simulink model "hummel_and_hubbard"  (R2021b)
settings: Solver=VariableStepAuto  StartTime=0.0  StopTime=10.0  RelTol=1e-3
values from neighbouring files (symbols this model uses):
  amb = evalin( 'base', 'amb')    [flatball_6dof_eqom.m]
  C = evalin( 'base', 'C')    [flatball_6dof_eqom.m]
  disc = evalin( 'base', 'disc')    [flatball_6dof_eqom.m]    (also in flatball_6dof_init.m = struct; flatball_init_disc_params.m = struct)
  Y0 = [0 0 -1, 0 15*C.DEG2RAD 0, 15 0 0, 0 0 (2*15*0.29/disc.d)]    [flatball_6dof_eqom.m]
libraries: simulink x4, aerolibanim x2, aerolibnav x2, matrix_library x2, mspfiltlib x1
(part 1 of 3)
settings Model: Creator=schae  LastModifiedBy=schae

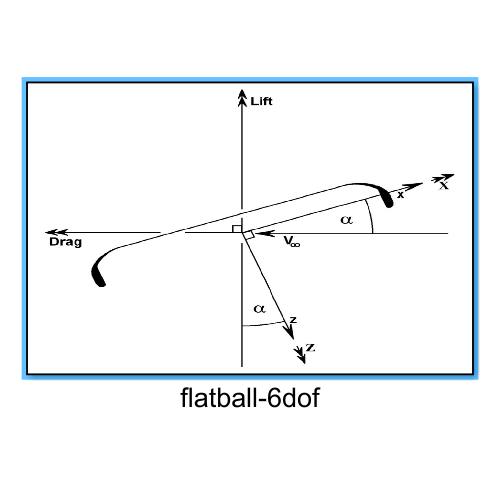
[thumbnail: Simulink's stored preview of the top-level diagram]
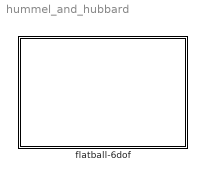
== system hummel_and_hubbard ==
  flatball-6dof : Subsystem
      mask Display: image('C:\.local\desktop\misc.protolabs\flatball-aero-ssl\arxiv\img\screenshots\flatball-6dof.png'); % Use "Edit Image" on toolstrip to change.

== system hummel_and_hubbard/flatball-6dof ==
  Integrator4 : Integrator  InitialConditionSource=external
  Selector : Selector  Commented=through  InputPortWidth=12  IndexOptions=Index vector (dialog)  Indices=[1 2 3 7 8 9 4 5 6 10 11 12]  OutputSizes=1
  Selector1 : Selector  Commented=through  InputPortWidth=12  IndexOptions=Index vector (dialog)  Indices=[1 2 3 7 8 9 4 5 6 10 11 12]  OutputSizes=1
  X0_desired : Constant  Value=Y0
  calc-F-M : Subsystem
  calc-Xdot : Subsystem
  lab : Subsystem
  wires:
  calc-F-M/2(M) -> [M]
  calc-F-M/1(F) -> [F]
  [X] -> Selector/1
  [F] -> calc-Xdot/2(F)
  calc-Xdot/1(Xdot) -> [dXdt], Integrator4/1
  X0_desired/1 -> Selector1/1
  [M] -> calc-Xdot/3(M)
  Integrator4/1 -> [X]  "X"
  [dXdt] -> lab/1(dYdt)
  [X] -> lab/2(Y)
  Selector/1 -> calc-F-M/1(X), calc-Xdot/1(X)
  Selector1/1 -> Integrator4/2

== system hummel_and_hubbard/flatball-6dof/calc-F-M ==
  X : Inport
  From1 : From  Commented=on  GotoTag=X
  From10 : From  Commented=on  GotoTag=F
  From11 : From  Commented=on  GotoTag=M
  From5 : From  Commented=on  GotoTag=alpha
  From6 : From  Commented=on  GotoTag=T
  From9 : From  Commented=on  GotoTag=wD
  calc-F : Subsystem
  calc-M : Subsystem
  calc-alpha : Subsystem
  lab : Subsystem  Commented=on
  rotations : Subsystem
  F : Outport
  M : Outport  Port=2
  wires:
  From1/1 -> lab/1(X)
  From10/1 -> lab/5(F)
  From6/1 -> lab/2(T)
  X/1 -> calc-M/1(X), calc-alpha/1(X), rotations/1(X), calc-F/1(X)
  [T] -> calc-M/2(T_c_N), calc-F/2(T_c_N)
  From9/1 -> lab/3(wD)
  [T] -> calc-alpha/2(T_c_N)
  rotations/1(T_c_N) -> [T]
  [alpha] -> calc-F/3(alpha), calc-M/4(alpha)
  From11/1 -> lab/6(M)
  rotations/2(wD_N) -> [wD]
  [wD] -> calc-M/3(wD_N_inN)
  calc-alpha/1(alpha) -> [alpha]
  From5/1 -> lab/4(alpha)
  calc-F/1(F) -> F/1  "F"
  calc-M/1(M) -> M/1  "M"

== system hummel_and_hubbard/flatball-6dof/calc-Xdot ==
  X : Inport
  F : Inport  Port=2
  M : Inport  Port=3
  Demux1 : Demux  Outputs=[1 1 1 1 1 1 1 1 1 1 1 1]
  Mux : Mux  Inputs=2
  Reshape : Reshape
  Selector : Selector  InputPortWidth=12  IndexOptions=Index vector (dialog)  Indices=[1 2 3 7 8 9 4 5 6 10 11 12]  OutputSizes=1
  Terminator{,1..11} (12 alike) : Terminator
  calc-THdot : MATLAB Function  TreatAsAtomicUnit=on
  calc-Xdot : MATLAB Function  TreatAsAtomicUnit=on
  Xdot : Outport
  wires:
  calc-Xdot/1(Xdot) -> Mux/1  "Xdot"
  Mux/1 -> Selector/1
  X/1 -> calc-THdot/1(X), calc-Xdot/1(X), [X]
  M/1 -> calc-THdot/2(M)
  F/1 -> calc-Xdot/2(F)
  calc-THdot/1(THdot) -> Mux/2  "THdot"
  Demux1/1 -> Terminator/1  "x"
  Demux1/2 -> Terminator1/1  "y"
  Demux1/3 -> Terminator2/1  "z"
  Demux1/6 -> Terminator5/1  "w"
  Demux1/5 -> Terminator4/1  "v"
  Demux1/4 -> Terminator3/1  "u"
  Demux1/10 -> Terminator9/1  "phidt"
  Demux1/11 -> Terminator10/1  "thetadt"
  Demux1/12 -> Terminator11/1  "psidt"
  Demux1/9 -> Terminator8/1  "psi"
  Demux1/8 -> Terminator7/1  "theta"
  Demux1/7 -> Terminator6/1  "phi"
  [X] -> Reshape/1
  Reshape/1 -> Demux1/1
  Selector/1 -> Xdot/1

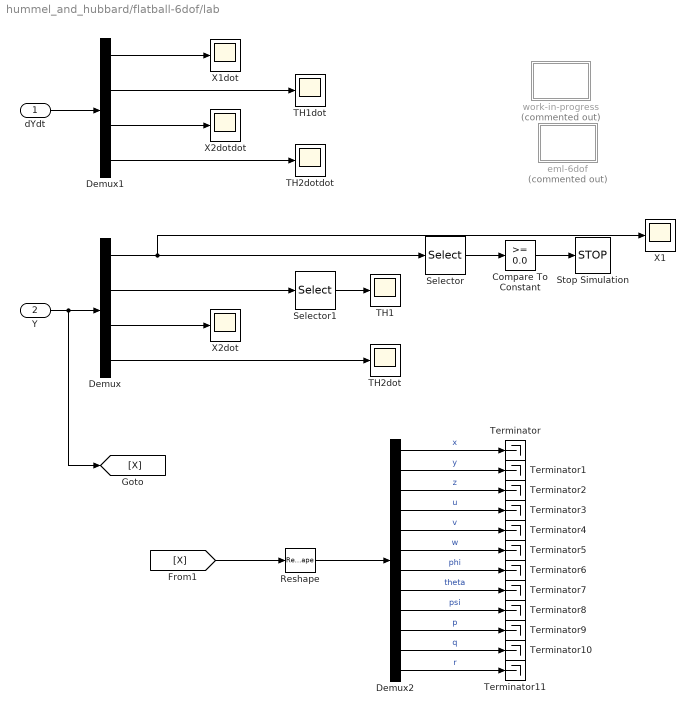
== system hummel_and_hubbard/flatball-6dof/lab ==
  dYdt : Inport
  Y : Inport  Port=2
  Compare To Constant : simulink/Logic and Bit Operations/Compare To Constant  relop=>=  const=0.0  OutDataTypeStr=boolean
  Demux : Demux  Outputs=[3 3 3 3]
  Demux1 : Demux  Outputs=[3 3 3 3]
  Demux2 : Demux  Outputs=[1 1 1 1 1 1 1 1 1 1 1 1]
  Reshape : Reshape
  Selector : Selector  InputPortWidth=3  IndexOptions=Index vector (dialog)  Indices=[3]  OutputSizes=1
  Selector1 : Selector  InputPortWidth=3  IndexOptions=Index vector (dialog)  Indices=[1 2]  OutputSizes=1
  Stop Simulation : Stop
  TH1 : Scope
  TH1dot : Scope
  TH2dot : Scope
  TH2dotdot : Scope
  Terminator{,1..11} (12 alike) : Terminator
  X1 : Scope
  X1dot : Scope
  X2dot : Scope
  X2dotdot : Scope
  eml-6dof : Subsystem  Commented=on
  work-in-progress : Subsystem  Commented=on
  wires:
  Demux2/4 -> Terminator3/1  "u"
  Demux2/3 -> Terminator2/1  "z"
  Demux2/2 -> Terminator1/1  "y"
  Demux2/6 -> Terminator5/1  "w"
  Demux2/1 -> Terminator/1  "x"
  Demux2/5 -> Terminator4/1  "v"
  Demux2/8 -> Terminator7/1  "theta"
  Demux2/7 -> Terminator6/1  "phi"
  Demux2/9 -> Terminator8/1  "psi"
  Demux2/10 -> Terminator9/1  "p"
  Demux2/11 -> Terminator10/1  "q"
  [X] -> Reshape/1
  Reshape/1 -> Demux2/1
  Demux2/12 -> Terminator11/1  "r"
  Compare To Constant/1 -> Stop Simulation/1
  Selector/1 -> Compare To Constant/1
  Selector1/1 -> TH1/1
  Y/1 -> Demux/1, [X]
  Demux/1 -> Selector/1, X1/1
  Demux/2 -> Selector1/1
  Demux/3 -> X2dot/1
  Demux/4 -> TH2dot/1
  dYdt/1 -> Demux1/1
  Demux1/1 -> X1dot/1
  Demux1/2 -> TH1dot/1
  Demux1/4 -> TH2dotdot/1
  Demux1/3 -> X2dotdot/1

== system hummel_and_hubbard/flatball-6dof/calc-F-M/calc-F ==
  X : Inport
  T_c_N : Inport  Port=2
  alpha : Inport  Port=3
  Fg_N : Constant  Value=[0 0 disc.m*amb.g]'
  Terminator{,1..3} (4 alike) : Terminator
  X-to-vel : MATLAB Function  TreatAsAtomicUnit=on
  aero-coeff : Subsystem
  calc-F : MATLAB Function  TreatAsAtomicUnit=on
  q-inf : Subsystem
  F : Outport
  wires:
  X-to-vel/1(vel) -> calc-F/1(vel)  "vel"
  X/1 -> q-inf/1(X), X-to-vel/1(X)
  T_c_N/1 -> calc-F/2(T_c_N)
  Fg_N/1 -> calc-F/3(Fg_N)
  calc-F/1(F) -> F/1  "F"
  q-inf/1(q-inf-S) -> calc-F/6(q_inf_times_S)
  alpha/1 -> aero-coeff/1(alpha)
  aero-coeff/1(Cl) -> calc-F/4(CLift)
  aero-coeff/2(Cd) -> calc-F/5(CDrag)
  q-inf/2(q-inf-S-d) -> Terminator/1
  calc-F/2(lift) -> Terminator1/1  "lift"
  calc-F/3(drag) -> Terminator2/1  "drag"
  calc-F/4(vmag) -> Terminator3/1  "v_inf"

== system hummel_and_hubbard/flatball-6dof/calc-F-M/calc-M ==
  X : Inport
  T_c_N : Inport  Port=2
  wD_N_inN : Inport  Port=3
  alpha : Inport  Port=4
  Terminator{,1..6} (7 alike) : Terminator
  X-to-vel : MATLAB Function  TreatAsAtomicUnit=on
  aero-coeff : Subsystem
  calc-M : MATLAB Function  TreatAsAtomicUnit=on
  internals : MATLAB Function  TreatAsAtomicUnit=on
  q-inf : Subsystem
  M : Outport
  wires:
  alpha/1 -> aero-coeff/1(alpha)
  calc-M/1(M) -> M/1  "M"
  T_c_N/1 -> calc-M/2(T_c_N), internals/2(T_c_N)
  X/1 -> X-to-vel/1(X), internals/1(X), q-inf/1(X)
  X-to-vel/1(vel) -> calc-M/1(vel)
  q-inf/2(q-inf-S-d) -> calc-M/4(q_inf_times_Sd)
  aero-coeff/1(Cm) -> calc-M/5(CMpitch)
  wD_N_inN/1 -> internals/3(wD_N_inN), calc-M/3(wD_N_inN)
  q-inf/1(q-inf-S) -> Terminator/1
  calc-M/2(p) -> Terminator1/1  "p"
  calc-M/3(q) -> Terminator2/1  "q"
  calc-M/4(r) -> Terminator3/1  "r"
  internals/3(E_rot) -> Terminator6/1  "E_rot"
  internals/2(E_trans) -> Terminator5/1  "E_trans"
  internals/1(AdvR) -> Terminator4/1  "AdvR"

== system hummel_and_hubbard/flatball-6dof/calc-F-M/calc-alpha ==
  X : Inport
  T_c_N : Inport  Port=2
  calc-alpha : MATLAB Function  TreatAsAtomicUnit=on
  alpha : Outport
  wires:
  calc-alpha/1(alpha) -> alpha/1  "alpha"
  X/1 -> calc-alpha/1(X)
  T_c_N/1 -> calc-alpha/2(T_c_N)

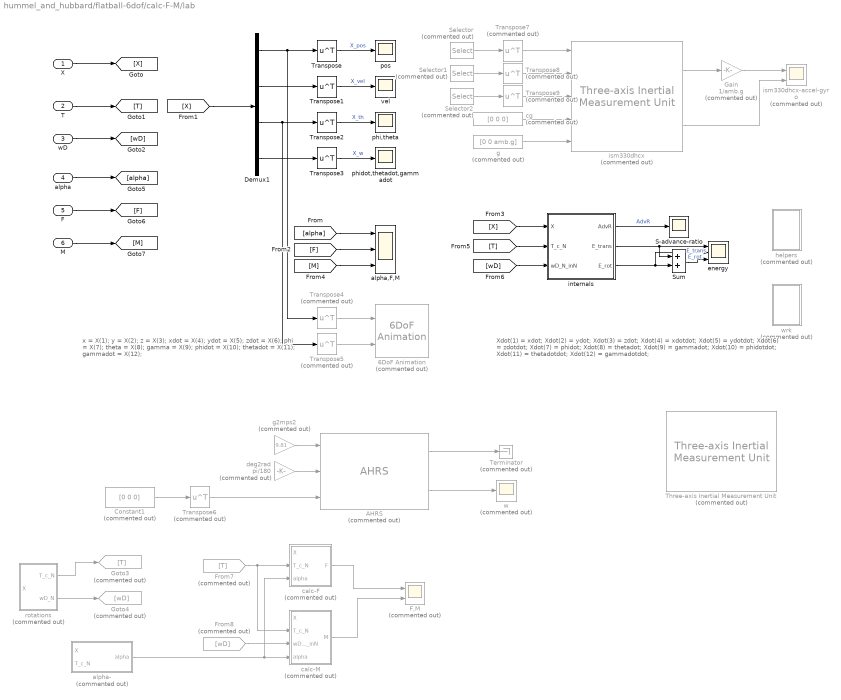
== system hummel_and_hubbard/flatball-6dof/calc-F-M/lab ==
  note: x = X(1); y = X(2); z = X(3);
      | xdot = X(4); ydot = X(5); zdot = X(6);
      |
      | phi = X(7); theta = X(8); gamma = X(9);
      | phidot = X(10); thetadot = X(11); gammadot = X(12);
  note: Xdot(1) = xdot; Xdot(2) = ydot; Xdot(3) = zdot;
      | Xdot(4) = xdotdot; Xdot(5) = ydotdot; Xdot(6) = zdotdot;
      |
      | Xdot(7) = phidot; Xdot(8) = thetadot; Xdot(9) = gammadot;
      | Xdot(10) = phidotdot; Xdot(11) = thetadotdot; Xdot(12) = gammadotdot;
  X : Inport
  T : Inport  Port=2
  wD : Inport  Port=3
  alpha : Inport  Port=4
  F : Inport  Port=5
  M : Inport  Port=6
  6DoF Animation : aerolibanim/6DoF Animation  Commented=on  u1=[-20 50 -20 50 -20 5]  u2=0.1  u3=1.0  u4=[-1 -1 -1]  u5=Fixed position  u6=[-200 -20 -10]  u7=10  u8=on
  AHRS : mspfiltlib/AHRS  Commented=on  DispRefFrame=ENU  DecimationFactor=1  InitialProcessNoise=ahrsfilter.defaultProcessNoise  OrientationFormat=Rotation matrix  SimulateUsing=Interpreted execution  AccelerometerNoise=0.0001924722  GyroscopeNoise=9.1385e-5  MagnetometerNoise=0.1  GyroscopeDriftNoise=3.0462e-13  LinearAccelerationNoise=0.0096236100000000012  MagneticDisturbanceNoise=0.5  LinearAccelerationDecayFactor=0.5  MagneticDisturbanceDecayFactor=0.5  ExpectedMagneticFieldStrength=50
      settings: SourceProductBaseCode=TF,NV
  Constant1 : Constant  Commented=on  Value=[0 0 0]
  Demux1 : Demux  Outputs=[3 3 3 3]
  F,M : Scope  Commented=on  NumInputPorts=2
  From7 : From  Commented=on  GotoTag=T
  From8 : From  Commented=on  GotoTag=wD
  Gain : Gain  Commented=on  Gain=1/amb.g
  Goto3 : Goto  Commented=on  GotoTag=T
  Goto4 : Goto  Commented=on  GotoTag=wD
  S-advance-ratio : Scope
  Selector : Selector  Commented=on  InputPortWidth=12  IndexOptions=Index vector (dialog)  Indices=[4 5 6]  OutputSizes=1
  Selector1 : Selector  Commented=on  InputPortWidth=12  IndexOptions=Index vector (dialog)  Indices=[7 8 9]  OutputSizes=1
  Selector2 : Selector  Commented=on  InputPortWidth=12  IndexOptions=Index vector (dialog)  Indices=[7 8 9]  OutputSizes=1
  Sum : Sum  Inputs=2
  Terminator : Terminator  Commented=on
  Three-axis Inertial Measurement Unit : aerolibnav/Three-axis Inertial Measurement Unit  Commented=on  units=Metric (MKS)  imu=[0 0 0]  i_Ts=0  dtype_a=on  w_a=190  z_a=0.707  a_sf_cc=[1 0 0; 0 1 0; 0 0 1]  a_bias=[0 0 0]  a_sat="[-inf  -inf  -inf  inf inf inf]"  dtype_g=on  w_g=190  z_g=0.707  g_sf_cc=[1 0 0; 0 1 0; 0 0 1]  g_bias=[0 0 0]  g_sens=[0 0 0]  g_sat="[-inf  -inf  -inf  inf inf inf]"  i_rand=on  i_seeds=[23093 23094 23095 23096 23097 23098]  i_pow=[0.001 0.001 0.001 0.0001 0.0001 0.0001]
  Transpose{,1..3} (4 alike) : Math  Operator=transpose  SaturateOnIntegerOverflow=on
  Transpose{4..9} (6 alike) : Math  Commented=on  Operator=transpose  SaturateOnIntegerOverflow=on
  alpha,F,M : Scope  NumInputPorts=3
  alpha- : MATLAB Function  Commented=on  TreatAsAtomicUnit=on
  calc-F : Subsystem  Commented=on
  calc-M : Subsystem  Commented=on
  cg : Constant  Commented=on  Value=[0 0 0]
  deg2rad : Gain  Commented=on  Gain=pi/180
  energy : Scope  NumInputPorts=3
  g : Constant  Commented=on  Value=[0 0 amb.g]
  g2mps2 : Gain  Commented=on  Gain=9.81
  helpers : Subsystem  Commented=on
  internals : MATLAB Function  TreatAsAtomicUnit=on
  ism330dhcx : aerolibnav/Three-axis Inertial Measurement Unit  Commented=on  units=Metric (MKS)  imu=[-2e-3 1e-3 -5e-3]  i_Ts=0  dtype_a=on  w_a=190  z_a=0.707  a_sf_cc=[1 0 0; 0 1 0; 0 0 1]  a_bias=[0 0 0]  a_sat="[-inf  -inf  -inf  inf inf inf]"  dtype_g=on  w_g=190  z_g=0.707  g_sf_cc=[1 0 0; 0 1 0; 0 0 1]  g_bias=[0 0 0]  g_sens=[0 0 0]  g_sat="[-inf  -inf  -inf  inf inf inf]"  i_rand=on  i_seeds=[23093 23094 23095 23096 23097 23098]  i_pow=[0.001 0.001 0.001 0.0001 0.0001 0.0001]
  ism330dhcx-accel-gyro : Scope  Commented=on  NumInputPorts=2
  phi,theta : Scope
  phidot,thetadot,gammadot : Scope
  pos : Scope
  rotations : Subsystem  Commented=on
  vel : Scope
  w : Scope  Commented=on
  wrk : Subsystem  Commented=on
  wires:
  From7/1 -> calc-M/2(T_c_N), calc-F/2(T_c_N)
  alpha-/1(alpha) -> calc-F/3(alpha), calc-M/4(alpha)
  From8/1 -> calc-M/3(wD_N_inN)
  calc-M/1(M) -> F,M/2
  calc-F/1(F) -> F,M/1
  rotations/1(T_c_N) -> Goto3/1
  rotations/2(wD_N) -> Goto4/1
  internals/3(E_rot) -> Sum/2, energy/2  "E_rot"
  [wD] -> internals/3(wD_N_inN)
  internals/1(AdvR) -> S-advance-ratio/1  "AdvR"
  [T] -> internals/2(T_c_N)
  Sum/1 -> energy/3
  [X] -> internals/1(X)
  internals/2(E_trans) -> Sum/1, energy/1  "E_trans"
  Demux1/4 -> Transpose3/1
  Demux1/3 -> Transpose5/1, Transpose2/1
  Demux1/1 -> Transpose4/1, Transpose/1
  Demux1/2 -> Transpose1/1
  [X] -> Demux1/1
  X/1 -> [X]
  T/1 -> [T]
  wD/1 -> [wD]
  F/1 -> [F]
  alpha/1 -> [alpha]
  M/1 -> [M]
  [alpha] -> alpha,F,M/1
  [F] -> alpha,F,M/2
  [M] -> alpha,F,M/3
  Transpose/1 -> pos/1  "X_pos"
  Transpose1/1 -> vel/1  "X_vel"
  Transpose2/1 -> phi,theta/1  "X_th"
  Transpose3/1 -> phidot,thetadot,gammadot/1  "X_w"
  Transpose4/1 -> 6DoF Animation/1
  Transpose5/1 -> 6DoF Animation/2
  Transpose6/1 -> AHRS/3
  Constant1/1 -> Transpose6/1
  AHRS/2 -> w/1
  g2mps2/1 -> AHRS/1
  deg2rad/1 -> AHRS/2
  AHRS/1 -> Terminator/1
  Transpose7/1 -> ism330dhcx/1
  Selector/1 -> Transpose7/1
  g/1 -> ism330dhcx/5
  Transpose8/1 -> ism330dhcx/2
  cg/1 -> ism330dhcx/4
  ism330dhcx/1 -> Gain/1
  Transpose9/1 -> ism330dhcx/3
  Selector1/1 -> Transpose8/1
  Selector2/1 -> Transpose9/1
  Gain/1 -> ism330dhcx-accel-gyro/1
  ism330dhcx/2 -> ism330dhcx-accel-gyro/2

== system hummel_and_hubbard/flatball-6dof/calc-F-M/rotations ==
  X : Inport
  MatrixMultiply3 : Product  Multiplication=Matrix(*)
  Transpose : Math  Operator=transpose  SaturateOnIntegerOverflow=on
  Transpose1 : Math  Operator=transpose  SaturateOnIntegerOverflow=on
  X-to-T_c_N : MATLAB Function  TreatAsAtomicUnit=on
  X-to-wD_N_inC : MATLAB Function  TreatAsAtomicUnit=on
  T_c_N : Outport
  wD_N : Outport  Port=2
  wires:
  X-to-T_c_N/1(T_c_N) -> Transpose1/1, T_c_N/1
  Transpose1/1 -> MatrixMultiply3/1
  X-to-wD_N_inC/1(wD_N_inC) -> Transpose/1
  Transpose/1 -> MatrixMultiply3/2
  MatrixMultiply3/1 -> wD_N/1
  X/1 -> X-to-wD_N_inC/1(X), X-to-T_c_N/1(X)

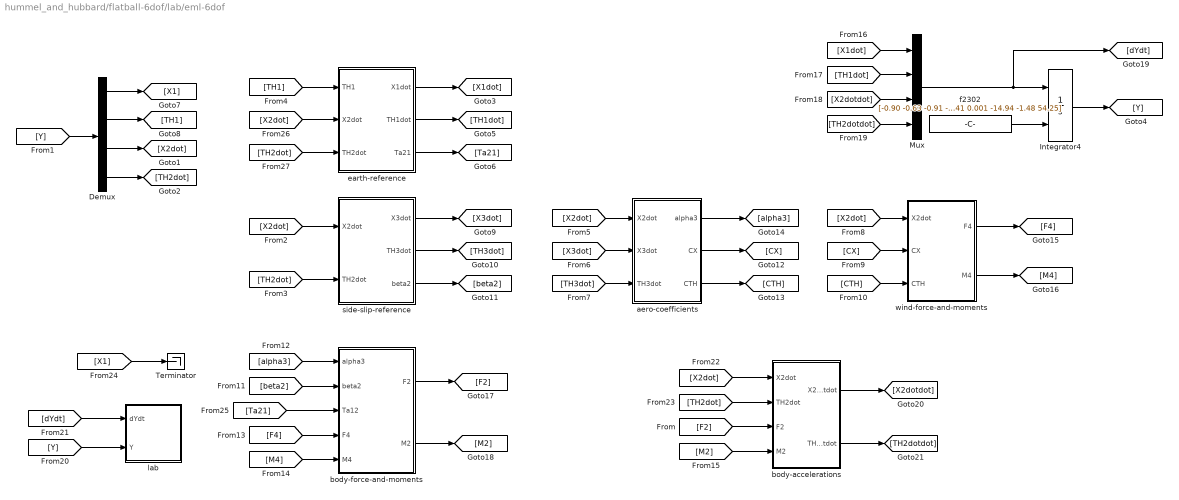
== system hummel_and_hubbard/flatball-6dof/lab/eml-6dof ==
  Demux : Demux  Outputs=[3 3 3 3]
  Integrator4 : Integrator  InitialConditionSource=external
  Mux : Mux
  Terminator : Terminator
  aero-coefficients : MATLAB Function  TreatAsAtomicUnit=on
  body-accelerations : MATLAB Function  TreatAsAtomicUnit=on
  body-force-and-moments : MATLAB Function  TreatAsAtomicUnit=on
  earth-reference : MATLAB Function  TreatAsAtomicUnit=on
  f2302 : Constant  Value=[-0.90 -0.63 -0.91 -0.07 0.21 5.03 13.42 -0.41 0.001 -14.94 -1.48 54.25]
  lab : Subsystem
  side-slip-reference : MATLAB Function  TreatAsAtomicUnit=on
  wind-force-and-moments : MATLAB Function  TreatAsAtomicUnit=on
  wires:
  earth-reference/1(X1dot) -> [X1dot]
  earth-reference/2(TH1dot) -> [TH1dot]
  earth-reference/3(Ta21) -> [Ta21]
  [Y] -> Demux/1
  Demux/1 -> [X1]
  Demux/2 -> [TH1]
  Demux/3 -> [X2dot]
  Demux/4 -> [TH2dot]
  [X2dot] -> side-slip-reference/1(X2dot)
  [TH2dot] -> side-slip-reference/2(TH2dot)
  side-slip-reference/1(X3dot) -> [X3dot]
  side-slip-reference/2(TH3dot) -> [TH3dot]
  side-slip-reference/3(beta2) -> [beta2]
  [TH1] -> earth-reference/1(TH1)
  [X2dot] -> aero-coefficients/1(X2dot)
  [X3dot] -> aero-coefficients/2(X3dot)
  [TH3dot] -> aero-coefficients/3(TH3dot)
  aero-coefficients/3(CTH) -> [CTH]
  aero-coefficients/2(CX) -> [CX]
  aero-coefficients/1(alpha3) -> [alpha3]
  [X2dot] -> wind-force-and-moments/1(X2dot)
  [CX] -> wind-force-and-moments/2(CX)
  [CTH] -> wind-force-and-moments/3(CTH)
  [beta2] -> body-force-and-moments/2(beta2)
  [alpha3] -> body-force-and-moments/1(alpha3)
  wind-force-and-moments/1(F4) -> [F4]
  wind-force-and-moments/2(M4) -> [M4]
  [F4] -> body-force-and-moments/4(F4)
  [M4] -> body-force-and-moments/5(M4)
  body-force-and-moments/1(F2) -> [F2]
  body-force-and-moments/2(M2) -> [M2]
  [TH2dotdot] -> Mux/4
  Mux/1 -> Integrator4/1, [dYdt]
  [TH1dot] -> Mux/2
  [X1dot] -> Mux/1
  f2302/1 -> Integrator4/2
  [X2dotdot] -> Mux/3
  Integrator4/1 -> [Y]
  [dYdt] -> lab/1(dYdt)
  [Y] -> lab/2(Y)
  [F2] -> body-accelerations/3(F2)
  [M2] -> body-accelerations/4(M2)
  [X2dot] -> body-accelerations/1(X2dot)
  [TH2dot] -> body-accelerations/2(TH2dot)
  body-accelerations/2(TH2dotdot) -> [TH2dotdot]
  body-accelerations/1(X2dotdot) -> [X2dotdot]
  [Ta21] -> body-force-and-moments/3(Ta12)
  [X1] -> Terminator/1
  [X2dot] -> earth-reference/2(X2dot)
  [TH2dot] -> earth-reference/3(TH2dot)

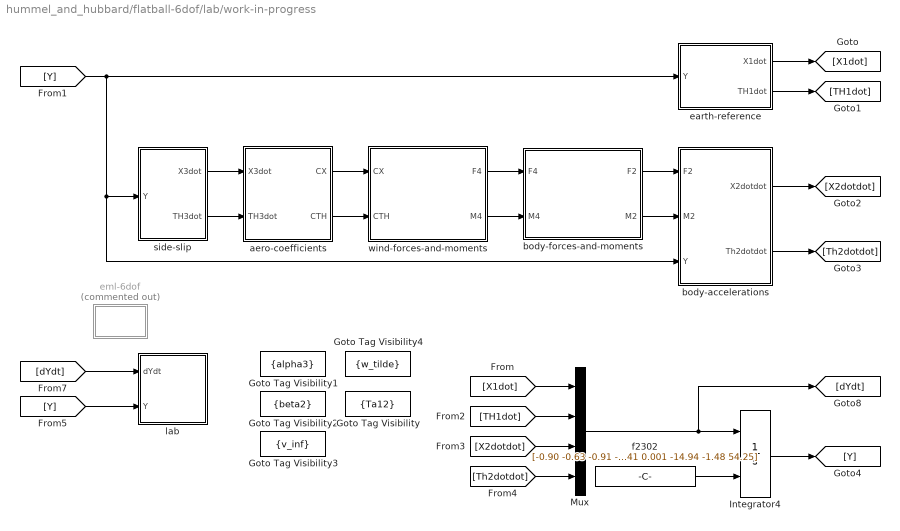
== system hummel_and_hubbard/flatball-6dof/lab/work-in-progress ==
  Goto Tag Visibility : GotoTagVisibility  GotoTag=Ta12
  Goto Tag Visibility1 : GotoTagVisibility  GotoTag=alpha3
  Goto Tag Visibility2 : GotoTagVisibility  GotoTag=beta2
  Goto Tag Visibility3 : GotoTagVisibility  GotoTag=v_inf
  Goto Tag Visibility4 : GotoTagVisibility  GotoTag=w_tilde
  Integrator4 : Integrator  InitialConditionSource=external
  Mux : Mux
  aero-coefficients : Subsystem
  body-accelerations : Subsystem
  body-forces-and-moments : Subsystem
  earth-reference : Subsystem
  eml-6dof : Subsystem  Commented=on
  f2302 : Constant  Value=[-0.90 -0.63 -0.91 -0.07 0.21 5.03 13.42 -0.41 0.001 -14.94 -1.48 54.25]
  lab : Subsystem
  side-slip : Subsystem
  wind-forces-and-moments : Subsystem
  wires:
  [X1dot] -> Mux/1
  [Y] -> lab/2(Y)
  [X2dotdot] -> Mux/3
  [Th2dotdot] -> Mux/4
  [dYdt] -> lab/1(dYdt)
  [TH1dot] -> Mux/2
  body-accelerations/1(X2dotdot) -> [X2dotdot]
  Mux/1 -> [dYdt], Integrator4/1
  Integrator4/1 -> [Y]
  [Y] -> earth-reference/1(Y), side-slip/1(Y), body-accelerations/3(Y)
  f2302/1 -> Integrator4/2
  body-accelerations/2(Th2dotdot) -> [Th2dotdot]
  earth-reference/2(TH1dot) -> [TH1dot]
  earth-reference/1(X1dot) -> [X1dot]
  body-forces-and-moments/2(M2) -> body-accelerations/2(M2)
  wind-forces-and-moments/2(M4) -> body-forces-and-moments/2(M4)
  wind-forces-and-moments/1(F4) -> body-forces-and-moments/1(F4)
  side-slip/2(TH3dot) -> aero-coefficients/2(TH3dot)
  body-forces-and-moments/1(F2) -> body-accelerations/1(F2)
  aero-coefficients/1(CX) -> wind-forces-and-moments/1(CX)
  side-slip/1(X3dot) -> aero-coefficients/1(X3dot)
  aero-coefficients/2(CTH) -> wind-forces-and-moments/2(CTH)

== system hummel_and_hubbard/flatball-6dof/calc-F-M/calc-F/aero-coeff ==
  alpha : Inport
  calc-Cd : Subsystem
  calc-Cl : Subsystem
  Cl : Outport
  Cd : Outport  Port=2
  wires:
  alpha/1 -> calc-Cl/1(alpha), calc-Cd/1(alpha)
  calc-Cl/1(Cl) -> Cl/1  "Cl"
  calc-Cd/1(Cd) -> Cd/1  "Cd"

== system hummel_and_hubbard/flatball-6dof/calc-F-M/calc-F/q-inf ==
  X : Inport
  Gain : Gain  Gain=0.5
  Product1 : Product  Inputs=3
  Product2 : Product
  S : Constant  Value=disc.A
  Square : Math  Operator=square  SaturateOnIntegerOverflow=on
  X-to-vel : MATLAB Function  TreatAsAtomicUnit=on
  d : Constant  Value=disc.d
  rho : Constant  Value=amb.rho
  vector-norm : MATLAB Function  TreatAsAtomicUnit=on
  q-inf-S : Outport
  q-inf-S-d : Outport  Port=2
  wires:
  Product1/1 -> Gain/1
  rho/1 -> Product1/3
  X/1 -> X-to-vel/1(X)
  vector-norm/1(norm) -> Square/1
  S/1 -> Product1/2
  Square/1 -> Product1/1
  Gain/1 -> Product2/1, q-inf-S/1
  X-to-vel/1(vel) -> vector-norm/1(vec)
  Product2/1 -> q-inf-S-d/1
  d/1 -> Product2/2

== system hummel_and_hubbard/flatball-6dof/calc-F-M/calc-M/aero-coeff ==
  alpha : Inport
  Subsystem2 : Subsystem
  Cm : Outport
  wires:
  alpha/1 -> Subsystem2/1(alpha)
  Subsystem2/1(Cm) -> Cm/1  "Cm"

== system hummel_and_hubbard/flatball-6dof/calc-F-M/calc-M/q-inf ==
  X : Inport
  Gain : Gain  Gain=0.5
  Product1 : Product  Inputs=3
  Product2 : Product
  S : Constant  Value=disc.A
  Square : Math  Operator=square  SaturateOnIntegerOverflow=on
  X-to-vel : MATLAB Function  TreatAsAtomicUnit=on
  d : Constant  Value=disc.d
  rho : Constant  Value=amb.rho
  vector-norm : MATLAB Function  TreatAsAtomicUnit=on
  q-inf-S : Outport
  q-inf-S-d : Outport  Port=2
  wires:
  d/1 -> Product2/2
  Product2/1 -> q-inf-S-d/1
  X-to-vel/1(vel) -> vector-norm/1(vec)
  Gain/1 -> q-inf-S/1, Product2/1
  Square/1 -> Product1/1
  S/1 -> Product1/2
  vector-norm/1(norm) -> Square/1
  X/1 -> X-to-vel/1(X)
  rho/1 -> Product1/3
  Product1/1 -> Gain/1

== system hummel_and_hubbard/flatball-6dof/calc-F-M/lab/calc-F ==
  X : Inport
  T_c_N : Inport  Port=2
  alpha : Inport  Port=3
  Fg_N : Constant  Value=[0 0 disc.m*amb.g]'
  Terminator : Terminator
  X-to-vel : MATLAB Function  TreatAsAtomicUnit=on
  aero-coeff : Subsystem
  calc-F : MATLAB Function  TreatAsAtomicUnit=on
  q-inf : Subsystem
  F : Outport
  wires:
  X-to-vel/1(vel) -> calc-F/1(vel)
  X/1 -> q-inf/1(X), X-to-vel/1(X)
  T_c_N/1 -> calc-F/2(T_c_N)
  Fg_N/1 -> calc-F/3(Fg_N)
  calc-F/1(F) -> F/1
  q-inf/1(q-inf-S) -> calc-F/6(q_inf_times_S)
  alpha/1 -> aero-coeff/1(alpha)
  aero-coeff/1(Cl) -> calc-F/4(CLift)
  aero-coeff/2(Cd) -> calc-F/5(CDrag)
  q-inf/2(q-inf-S-d) -> Terminator/1

== system hummel_and_hubbard/flatball-6dof/calc-F-M/lab/calc-M ==
  X : Inport
  T_c_N : Inport  Port=2
  wD_N_inN : Inport  Port=3
  alpha : Inport  Port=4
  Terminator : Terminator
  X-to-vel : MATLAB Function  TreatAsAtomicUnit=on
  aero-coeff : Subsystem
  calc-M : MATLAB Function  TreatAsAtomicUnit=on
  q-inf : Subsystem
  M : Outport
  wires:
  alpha/1 -> aero-coeff/1(alpha)
  calc-M/1(M) -> M/1
  T_c_N/1 -> calc-M/2(T_c_N)
  X/1 -> X-to-vel/1(X), q-inf/1(X)
  X-to-vel/1(vel) -> calc-M/1(vel)
  q-inf/2(q-inf-S-d) -> calc-M/5(q_inf_times_Sd)
  aero-coeff/1(Cm) -> calc-M/4(CMpitch)
  wD_N_inN/1 -> calc-M/3(wD_N_inN)
  q-inf/1(q-inf-S) -> Terminator/1

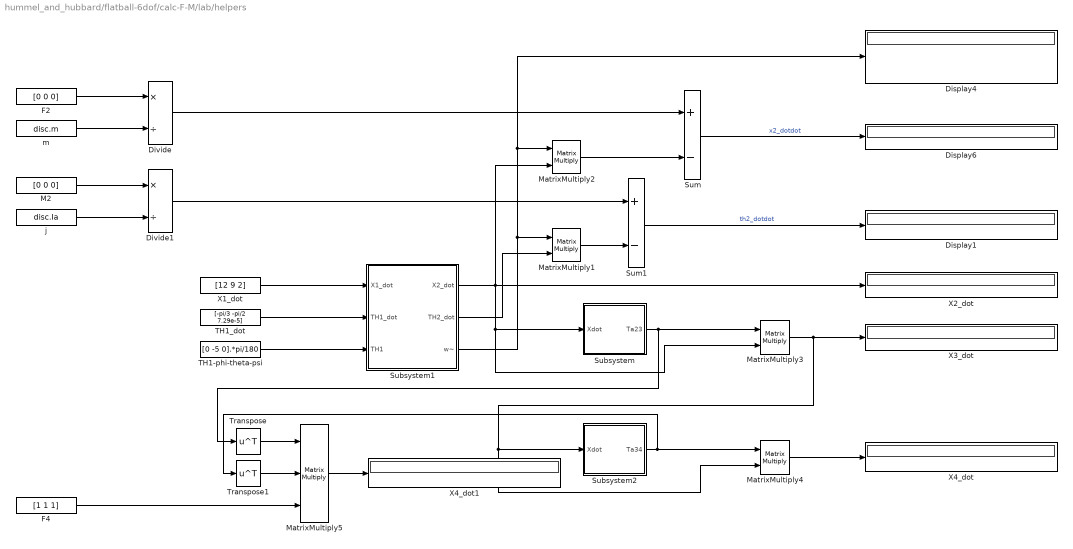
== system hummel_and_hubbard/flatball-6dof/calc-F-M/lab/helpers ==
  Display1 : Display
  Display4 : Display
  Display6 : Display
  Divide : Product  Inputs=*/
  Divide1 : Product  Inputs=*/
  F2 : Constant  Value=[0 0 0]
  F4 : Constant  Value=[1 1 1]
  M2 : Constant  Value=[0 0 0]
  MatrixMultiply{1..4} (4 alike) : Product  Multiplication=Matrix(*)
  MatrixMultiply5 : Product  Inputs=***  Multiplication=Matrix(*)
  Subsystem : Subsystem
  Subsystem1 : Subsystem
  Subsystem2 : Subsystem
  Sum : Sum  Inputs=+-
  Sum1 : Sum  Inputs=+-
  TH1-phi-theta-psi : Constant  Value=[0 -5 0].*pi/180
  TH1_dot : Constant  Value=[-pi/3 -pi/2 7.29e-5]
  Transpose : Math  Operator=transpose  SaturateOnIntegerOverflow=on
  Transpose1 : Math  Operator=transpose  SaturateOnIntegerOverflow=on
  X1_dot : Constant  Value=[12 9 2]
  X2_dot : Display
  X3_dot : Display
  X4_dot : Display
  X4_dot1 : Display
  j : Constant  Value=disc.Ia
  m : Constant  Value=disc.m
  wires:
  X1_dot/1 -> Subsystem1/1(X1_dot)
  TH1_dot/1 -> Subsystem1/2(TH1_dot)
  TH1-phi-theta-psi/1 -> Subsystem1/3(TH1)
  MatrixMultiply2/1 -> Sum/2
  Subsystem1/3(w~) -> MatrixMultiply1/1, Display4/1, MatrixMultiply2/1
  Subsystem1/1(X2_dot) -> MatrixMultiply2/2, X2_dot/1, MatrixMultiply3/2, Subsystem/1(Xdot)
  F2/1 -> Divide/1
  m/1 -> Divide/2
  Divide/1 -> Sum/1
  Sum/1 -> Display6/1  "x2_dotdot"
  j/1 -> Divide1/2
  M2/1 -> Divide1/1
  Divide1/1 -> Sum1/1
  MatrixMultiply1/1 -> Sum1/2
  Subsystem1/2(TH2_dot) -> MatrixMultiply1/2
  Sum1/1 -> Display1/1  "th2_dotdot"
  Subsystem/1(Ta23) -> Transpose/1, MatrixMultiply3/1
  MatrixMultiply3/1 -> MatrixMultiply4/2, Subsystem2/1(Xdot), X3_dot/1
  Subsystem2/1(Ta34) -> Transpose1/1, MatrixMultiply4/1
  MatrixMultiply4/1 -> X4_dot/1
  Transpose1/1 -> MatrixMultiply5/2
  Transpose/1 -> MatrixMultiply5/1
  F4/1 -> MatrixMultiply5/3
  MatrixMultiply5/1 -> X4_dot1/1

== system hummel_and_hubbard/flatball-6dof/calc-F-M/lab/rotations ==
  X : Inport
  MatrixMultiply3 : Product  Multiplication=Matrix(*)
  Transpose : Math  Operator=transpose  SaturateOnIntegerOverflow=on
  Transpose1 : Math  Operator=transpose  SaturateOnIntegerOverflow=on
  X-to-T_c_N : MATLAB Function  TreatAsAtomicUnit=on
  X-to-wD_N_inC : MATLAB Function  TreatAsAtomicUnit=on
  T_c_N : Outport
  wD_N : Outport  Port=2
  wires:
  X-to-T_c_N/1(T_c_N) -> Transpose1/1, T_c_N/1
  Transpose1/1 -> MatrixMultiply3/1
  X-to-wD_N_inC/1(wD_N_inC) -> Transpose/1
  Transpose/1 -> MatrixMultiply3/2
  MatrixMultiply3/1 -> wD_N/1
  X/1 -> X-to-wD_N_inC/1(X), X-to-T_c_N/1(X)

== system hummel_and_hubbard/flatball-6dof/calc-F-M/lab/wrk ==
  6DoF Animation : aerolibanim/6DoF Animation  Commented=on  u1=[-10 100 -20 100 -10 10]  u2=0.01  u3=5  u4=[1 0 -5]  u5=Fixed position  u6=[100 50 -500]  u7=10  u8=on
  Demux : Demux  Commented=on  Outputs=[3 3 3 3]
  From : From  Commented=on  GotoTag=x1
  From1 : From  Commented=on  GotoTag=x1dt
  From2 : From  Commented=on  GotoTag=theta1
  From3 : From  Commented=on  GotoTag=theta1dt
  From5 : From  Commented=on  GotoTag=theta1
  From6 : From  Commented=on  GotoTag=theta1dt
  From7 : From  Commented=on  GotoTag=x1dt
  Transpose{3..6} (4 alike) : Math  Commented=on  Operator=transpose  SaturateOnIntegerOverflow=on
  c&p : Subsystem  Commented=on
  flatball_6dof : MATLAB Function  Commented=on  TreatAsAtomicUnit=on
  flatball_6dof_v1p0 : MATLAB Function  Commented=on  TreatAsAtomicUnit=on
  flatball_6dof_v1p1 : MATLAB Function  Commented=on  TreatAsAtomicUnit=on
  hummel : Subsystem  Commented=on
  wires:
  From/1 -> Transpose3/1
  From2/1 -> Transpose5/1
  From3/1 -> Transpose6/1
  Demux/3 -> 6DoF Animation/2
  Transpose3/1 -> c&p/1(x1)
  Demux/1 -> 6DoF Animation/1
  From1/1 -> Transpose4/1
  Transpose5/1 -> c&p/3(theta1)
  Transpose4/1 -> c&p/2(x1dt)
  Transpose6/1 -> c&p/4(theta1dt)
  From5/1 -> hummel/2(TH)
  From6/1 -> hummel/3(TH-dt)
  From7/1 -> hummel/1(vel)

== system hummel_and_hubbard/flatball-6dof/lab/eml-6dof/lab ==
  dYdt : Inport
  Y : Inport  Port=2
  Compare To Constant : simulink/Logic and Bit Operations/Compare To Constant  relop=>=  const=0.0  OutDataTypeStr=boolean
  Demux : Demux  Outputs=[3 3 3 3]
  Demux1 : Demux  Outputs=[3 3 3 3]
  Selector : Selector  InputPortWidth=3  IndexOptions=Index vector (dialog)  Indices=[3]  OutputSizes=1
  Selector1 : Selector  InputPortWidth=3  IndexOptions=Index vector (dialog)  Indices=[1 2]  OutputSizes=1
  Stop Simulation : Stop
  TH1 : Scope
  TH1dot : Scope
  TH2dot : Scope
  TH2dotdot : Scope
  X1 : Scope
  X1dot : Scope
  X2dot : Scope
  X2dotdot : Scope
  wires:
  Compare To Constant/1 -> Stop Simulation/1
  Selector/1 -> Compare To Constant/1
  Selector1/1 -> TH1/1
  Y/1 -> Demux/1
  Demux/1 -> Selector/1, X1/1
  Demux/2 -> Selector1/1
  Demux/3 -> X2dot/1
  Demux/4 -> TH2dot/1
  dYdt/1 -> Demux1/1
  Demux1/1 -> X1dot/1
  Demux1/2 -> TH1dot/1
  Demux1/4 -> TH2dotdot/1
  Demux1/3 -> X2dotdot/1

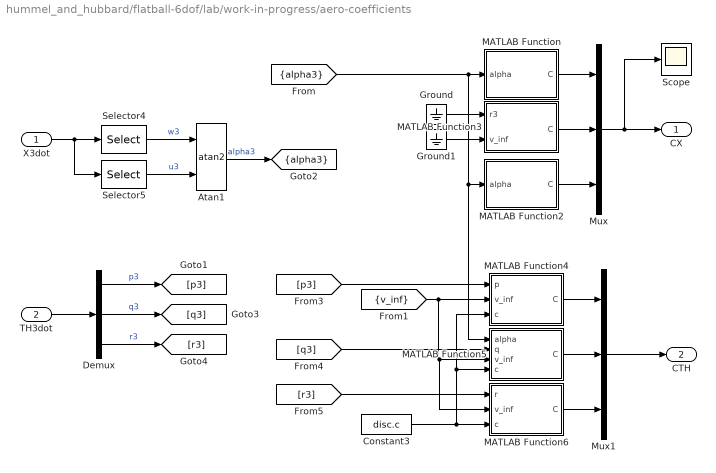
== system hummel_and_hubbard/flatball-6dof/lab/work-in-progress/aero-coefficients ==
  X3dot : Inport
  TH3dot : Inport  Port=2
  Atan1 : Trigonometry  Operator=atan2
  Constant3 : Constant  Value=disc.c
  Demux : Demux  Outputs=3
  Ground : Ground
  Ground1 : Ground
  MATLAB Function : MATLAB Function  TreatAsAtomicUnit=on
  MATLAB Function2 : MATLAB Function  TreatAsAtomicUnit=on
  MATLAB Function3 : MATLAB Function  TreatAsAtomicUnit=on
  MATLAB Function4 : MATLAB Function  TreatAsAtomicUnit=on
  MATLAB Function5 : MATLAB Function  TreatAsAtomicUnit=on
  MATLAB Function6 : MATLAB Function  TreatAsAtomicUnit=on
  Mux : Mux  Inputs=3
  Mux1 : Mux  Inputs=3
  Scope : Scope
  Selector4 : Selector  InputPortWidth=3  IndexOptions=Index vector (dialog)  Indices=[3]  OutputSizes=1
  Selector5 : Selector  InputPortWidth=3  IndexOptions=Index vector (dialog)  Indices=[1]  OutputSizes=1
  CX : Outport
  CTH : Outport  Port=2
  tag scope: alpha3=scoped
  wires:
  Ground1/1 -> MATLAB Function3/2(v_inf)
  Ground/1 -> MATLAB Function3/1(r3)
  TH3dot/1 -> Demux/1
  [r3] -> MATLAB Function6/1(r)
  [q3] -> MATLAB Function5/2(q)
  [p3] -> MATLAB Function4/1(p)
  [v_inf] -> MATLAB Function4/2(v_inf), MATLAB Function5/3(v_inf), MATLAB Function6/2(v_inf)
  Constant3/1 -> MATLAB Function6/3(c), MATLAB Function5/4(c), MATLAB Function4/3(c)
  [alpha3] -> MATLAB Function/1(alpha), MATLAB Function5/1(alpha), MATLAB Function2/1(alpha)
  Mux1/1 -> CTH/1
  Mux/1 -> CX/1, Scope/1
  MATLAB Function4/1(C) -> Mux1/1
  MATLAB Function5/1(C) -> Mux1/2
  MATLAB Function6/1(C) -> Mux1/3
  MATLAB Function/1(C) -> Mux/1
  MATLAB Function2/1(C) -> Mux/3
  MATLAB Function3/1(C) -> Mux/2
  X3dot/1 -> Selector4/1, Selector5/1
  Demux/3 -> [r3]  "r3"
  Demux/2 -> [q3]  "q3"
  Demux/1 -> [p3]  "p3"
  Atan1/1 -> [alpha3]  "alpha3"
  Selector4/1 -> Atan1/1  "w3"
  Selector5/1 -> Atan1/2  "u3"

== system hummel_and_hubbard/flatball-6dof/lab/work-in-progress/body-accelerations ==
  F2 : Inport
  M2 : Inport  Port=2
  Y : Inport  Port=3
  Constant1 : Constant  Value=disc.I
  Constant2 : Constant  Value=disc.m
  Constant3 : Constant  Value=disc.I ^ -1
  Product : Product  Multiplication=Matrix(*)
  Product1 : Product  Inputs=*/
  Product4 : Product  Inputs=3  Multiplication=Matrix(*)
  Product5 : Product  Multiplication=Matrix(*)
  Sum : Sum  Inputs=+-
  Sum1 : Sum  Inputs=+-
  TH2dot : Selector  InputPortWidth=12  IndexOptions=Index vector (dialog)  Indices=[10 11 12]  OutputSizes=1
  X2dot : Selector  InputPortWidth=12  IndexOptions=Index vector (dialog)  Indices=[7 8 9]  OutputSizes=1
  X2dotdot : Outport
  Th2dotdot : Outport  Port=2
  wires:
  TH2dot/1 -> Product4/3
  Constant1/1 -> Product4/2
  [w_tilde] -> Product4/1
  [w_tilde] -> Product/1
  Y/1 -> TH2dot/1, X2dot/1
  Product5/1 -> Th2dotdot/1
  Constant3/1 -> Product5/1
  Sum1/1 -> Product5/2
  Product4/1 -> Sum1/2
  M2/1 -> Sum1/1
  Sum/1 -> X2dotdot/1
  Product/1 -> Sum/2
  Product1/1 -> Sum/1
  Constant2/1 -> Product1/2
  F2/1 -> Product1/1
  X2dot/1 -> Product/2

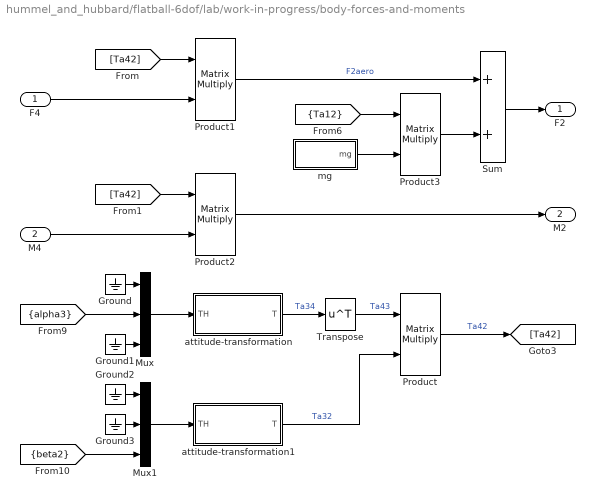
== system hummel_and_hubbard/flatball-6dof/lab/work-in-progress/body-forces-and-moments ==
  F4 : Inport
  M4 : Inport  Port=2
  Ground{,1..3} (4 alike) : Ground
  Mux : Mux  Inputs=3
  Mux1 : Mux  Inputs=3
  Product{,1..3} (4 alike) : Product  Multiplication=Matrix(*)
  Sum : Sum
  Transpose : Math  Operator=transpose  SaturateOnIntegerOverflow=on
  attitude-transformation : MATLAB Function  TreatAsAtomicUnit=on
  attitude-transformation1 : MATLAB Function  TreatAsAtomicUnit=on
  mg : Subsystem
  F2 : Outport
  M2 : Outport  Port=2
  wires:
  [Ta12] -> Product3/1
  [alpha3] -> Mux/2
  [beta2] -> Mux1/3
  mg/1(mg) -> Product3/2
  Sum/1 -> F2/1
  Product3/1 -> Sum/2
  Product2/1 -> M2/1
  Product1/1 -> Sum/1  "F2aero"
  [Ta42] -> Product2/1
  M4/1 -> Product2/2
  F4/1 -> Product1/2
  [Ta42] -> Product1/1
  Product/1 -> [Ta42]  "Ta42"
  attitude-transformation/1(T) -> Transpose/1  "Ta34"
  Transpose/1 -> Product/1  "Ta43"
  attitude-transformation1/1(T) -> Product/2  "Ta32"
  Ground2/1 -> Mux1/1
  Ground3/1 -> Mux1/2
  Mux1/1 -> attitude-transformation1/1(TH)
  Mux/1 -> attitude-transformation/1(TH)
  Ground/1 -> Mux/1
  Ground1/1 -> Mux/3

== system hummel_and_hubbard/flatball-6dof/lab/work-in-progress/earth-reference ==
  Y : Inport
  Product : Product  Multiplication=Matrix(*)
  Product1 : Product  Multiplication=Matrix(*)
  TH1 : Selector  InputPortWidth=12  IndexOptions=Index vector (dialog)  Indices=[4 5 6]  OutputSizes=1
  TH2dot : Selector  InputPortWidth=12  IndexOptions=Index vector (dialog)  Indices=[10 11 12]  OutputSizes=1
  Transpose : Math  Operator=transpose  SaturateOnIntegerOverflow=on
  X2dot : Selector  InputPortWidth=12  IndexOptions=Index vector (dialog)  Indices=[7 8 9]  OutputSizes=1
  attitude-transformation : MATLAB Function  TreatAsAtomicUnit=on
  beta2 : Subsystem
  rate-transformation : MATLAB Function  TreatAsAtomicUnit=on
  v_inf : Subsystem
  w_tilde : Subsystem
  X1dot : Outport
  TH1dot : Outport  Port=2
  tag scope: Ta12=scoped
  wires:
  Transpose/1 -> [Ta12]
  [Ta21] -> Transpose/1
  Product1/1 -> TH1dot/1
  Product/1 -> X1dot/1
  [Tr21] -> Product1/1
  TH2dot/1 -> Product1/2  "TH2dot"
  X2dot/1 -> beta2/1(X2dot), v_inf/1(X2dot), w_tilde/1(X2dot), Product/2  "X2dot"
  [Ta21] -> Product/1
  rate-transformation/1(T) -> [Tr21]
  Y/1 -> TH2dot/1, X2dot/1, TH1/1
  attitude-transformation/1(T) -> [Ta21]
  TH1/1 -> rate-transformation/1(TH), attitude-transformation/1(TH)  "TH1"

== system hummel_and_hubbard/flatball-6dof/lab/work-in-progress/eml-6dof ==
  Integrator4 : Integrator  InitialConditionSource=external
  MATLAB Function : MATLAB Function  TreatAsAtomicUnit=on
  f2302 : Constant  Value=[-0.90 -0.63 -0.91 -0.07 0.21 5.03 13.42 -0.41 0.001 -14.94 -1.48 54.25]
  lab : Subsystem
  wires:
  MATLAB Function/11(dydt) -> Integrator4/1
  MATLAB Function/9(alpha3) -> lab/9(alpha3)
  MATLAB Function/8(TH3dot) -> lab/8(TH3-dot)
  Integrator4/1 -> [X]  "X"
  MATLAB Function/1(X1) -> lab/1(X1)
  f2302/1 -> Integrator4/2, MATLAB Function/2(X0)
  [X] -> MATLAB Function/1(X)
  MATLAB Function/2(TH1) -> lab/2(TH1)
  MATLAB Function/5(X2dot) -> lab/5(X2-dot)
  MATLAB Function/6(TH2dot) -> lab/6(TH2-dot)
  MATLAB Function/4(TH1dot) -> lab/4(TH1-dot)
  MATLAB Function/10(beta2) -> lab/10(beta2)
  MATLAB Function/3(X1dot) -> lab/3(X1-dot)
  MATLAB Function/7(X3dot) -> lab/7(X3-dot)

== system hummel_and_hubbard/flatball-6dof/lab/work-in-progress/lab ==
  dYdt : Inport
  Y : Inport  Port=2
  Compare To Constant : simulink/Logic and Bit Operations/Compare To Constant  relop=>=  const=0.0  OutDataTypeStr=boolean
  Demux : Demux  Outputs=[3 3 3 3]
  Demux1 : Demux  Outputs=[3 3 3 3]
  Gain : Gain  Gain=C.RAD2DEG
  Gain1 : Gain  Gain=C.RAD2DEG
  Scope1 : Scope
  Scope9 : Scope
  Selector : Selector  InputPortWidth=3  IndexOptions=Index vector (dialog)  Indices=[3]  OutputSizes=1
  Selector1 : Selector  InputPortWidth=3  IndexOptions=Index vector (dialog)  Indices=[1 2]  OutputSizes=1
  Stop Simulation : Stop
  TH1 : Scope
  TH1dot : Scope
  TH2dot : Scope
  TH2dotdot : Scope
  X1 : Scope
  X1dot : Scope
  X2dot : Scope
  X2dotdot : Scope
  wires:
  [beta2] -> Gain1/1
  [alpha3] -> Gain/1
  Demux1/3 -> X2dotdot/1
  Demux1/4 -> TH2dotdot/1
  Demux1/2 -> TH1dot/1
  Demux1/1 -> X1dot/1
  dYdt/1 -> Demux1/1
  Demux/4 -> TH2dot/1
  Demux/3 -> X2dot/1
  Demux/2 -> Selector1/1
  Demux/1 -> X1/1, Selector/1
  Y/1 -> Demux/1
  Selector1/1 -> TH1/1
  Gain1/1 -> Scope9/1
  Gain/1 -> Scope1/1
  Selector/1 -> Compare To Constant/1
  Compare To Constant/1 -> Stop Simulation/1

== system hummel_and_hubbard/flatball-6dof/lab/work-in-progress/side-slip ==
  Y : Inport
  Ground : Ground
  Ground1 : Ground
  Mux : Mux  Inputs=3
  Product : Product  Multiplication=Matrix(*)
  Product1 : Product  Multiplication=Matrix(*)
  TH2dot : Selector  InputPortWidth=12  IndexOptions=Index vector (dialog)  Indices=[10 11 12]  OutputSizes=1
  Transpose : Math  Operator=transpose  SaturateOnIntegerOverflow=on
  X2dot : Selector  InputPortWidth=12  IndexOptions=Index vector (dialog)  Indices=[7 8 9]  OutputSizes=1
  attitude-transformation : MATLAB Function  TreatAsAtomicUnit=on
  X3dot : Outport
  TH3dot : Outport  Port=2
  wires:
  Transpose/1 -> [Ta23]  "Ta23"
  Ground1/1 -> Mux/2
  Ground/1 -> Mux/1
  attitude-transformation/1(T) -> Transpose/1  "Ta32"
  Mux/1 -> attitude-transformation/1(TH)
  [beta2] -> Mux/3
  Y/1 -> X2dot/1, TH2dot/1
  [Ta23] -> Product/1, Product1/1  "Ta23"
  X2dot/1 -> Product/2  "X2dot"
  TH2dot/1 -> Product1/2  "TH2dot"
  Product/1 -> X3dot/1
  Product1/1 -> TH3dot/1

== system hummel_and_hubbard/flatball-6dof/lab/work-in-progress/wind-forces-and-moments ==
  CX : Inport
  CTH : Inport  Port=2
  Constant : Constant  Value=amb.rho / 2
  Constant1 : Constant  Value=disc.S
  Constant2 : Constant  Value=disc.c
  Demux : Demux  Outputs=3
  Gain : Gain  Gain=-1
  Gain1 : Gain  Gain=0
  Gain2 : Gain  Gain=-1
  Mux : Mux  Inputs=3
  Product1 : Product  Inputs=3
  Product2 : Product
  Product3 : Product
  Product4 : Product
  Square : Math  Operator=square  SaturateOnIntegerOverflow=on
  F4 : Outport
  M4 : Outport  Port=2
  wires:
  Constant2/1 -> Product1/3
  Product3/1 -> [qS]
  Square/1 -> Product4/2
  [v_inf] -> Square/1
  Product4/1 -> Product3/1  "q_inf"
  Constant/1 -> Product4/1
  Constant1/1 -> Product3/2
  Mux/1 -> Product2/1
  Gain2/1 -> Mux/3
  Gain/1 -> Mux/1
  Gain1/1 -> Mux/2
  Demux/3 -> Gain2/1
  Demux/2 -> Gain1/1
  Demux/1 -> Gain/1
  CX/1 -> Demux/1
  [qS] -> Product2/2, Product1/2
  CTH/1 -> Product1/1
  Product2/1 -> F4/1
  Product1/1 -> M4/1

== system hummel_and_hubbard/flatball-6dof/calc-F-M/calc-F/aero-coeff/calc-Cd ==
  alpha : Inport
  Cd0 : Constant  Value=disc.CD0
  Cda : Constant  Value=disc.CDa
  Product : Product
  Square : Math  Operator=square  SaturateOnIntegerOverflow=on
  Sum : Sum  Inputs=+-
  Sum1 : Sum
  alpha0 : Constant  Value=disc.alpha0
  Cd : Outport
  wires:
  Sum1/1 -> Cd/1
  Square/1 -> Product/2
  Product/1 -> Sum1/2
  Cda/1 -> Product/1
  Cd0/1 -> Sum1/1
  Sum/1 -> Square/1
  alpha0/1 -> Sum/2
  alpha/1 -> Sum/1

== system hummel_and_hubbard/flatball-6dof/calc-F-M/calc-F/aero-coeff/calc-Cl ==
  alpha : Inport
  CL0 : Constant  Value=disc.CL0
  CLa : Constant  Value=disc.CLa
  Product : Product
  Sum1 : Sum
  Cl : Outport
  wires:
  alpha/1 -> Product/2
  CL0/1 -> Sum1/1
  CLa/1 -> Product/1
  Product/1 -> Sum1/2
  Sum1/1 -> Cl/1

== system hummel_and_hubbard/flatball-6dof/calc-F-M/calc-M/aero-coeff/Subsystem2 ==
  alpha : Inport
  CM0 : Constant  Value=disc.CM0
  CMa : Constant  Value=disc.CMa
  Product : Product
  Sum1 : Sum
  Cm : Outport
  wires:
  Sum1/1 -> Cm/1
  Product/1 -> Sum1/2
  CMa/1 -> Product/1
  CM0/1 -> Sum1/1
  alpha/1 -> Product/2

== system hummel_and_hubbard/flatball-6dof/calc-F-M/lab/calc-F/aero-coeff ==
  alpha : Inport
  Subsystem : Subsystem
  Subsystem1 : Subsystem
  Cl : Outport
  Cd : Outport  Port=2
  wires:
  alpha/1 -> Subsystem1/1(alpha), Subsystem/1(alpha)
  Subsystem1/1(Cl) -> Cl/1
  Subsystem/1(Cd) -> Cd/1

== system hummel_and_hubbard/flatball-6dof/calc-F-M/lab/calc-F/q-inf ==
  X : Inport
  Gain : Gain  Gain=0.5
  Product1 : Product  Inputs=3
  Product2 : Product
  S : Constant  Value=disc.A
  Square : Math  Operator=square  SaturateOnIntegerOverflow=on
  X-to-vel : MATLAB Function  TreatAsAtomicUnit=on
  d : Constant  Value=disc.d
  rho : Constant  Value=amb.rho
  vector-norm : MATLAB Function  TreatAsAtomicUnit=on
  q-inf-S : Outport
  q-inf-S-d : Outport  Port=2
  wires:
  Product1/1 -> Gain/1
  rho/1 -> Product1/3
  X/1 -> X-to-vel/1(X)
  vector-norm/1(norm) -> Square/1
  S/1 -> Product1/2
  Square/1 -> Product1/1
  Gain/1 -> Product2/1, q-inf-S/1
  X-to-vel/1(vel) -> vector-norm/1(vec)
  Product2/1 -> q-inf-S-d/1
  d/1 -> Product2/2

== system hummel_and_hubbard/flatball-6dof/calc-F-M/lab/calc-M/aero-coeff ==
  alpha : Inport
  Subsystem2 : Subsystem
  Cm : Outport
  wires:
  alpha/1 -> Subsystem2/1(alpha)
  Subsystem2/1(Cm) -> Cm/1

== system hummel_and_hubbard/flatball-6dof/calc-F-M/lab/calc-M/q-inf ==
  X : Inport
  Gain : Gain  Gain=0.5
  Product1 : Product  Inputs=3
  Product2 : Product
  S : Constant  Value=disc.A
  Square : Math  Operator=square  SaturateOnIntegerOverflow=on
  X-to-vel : MATLAB Function  TreatAsAtomicUnit=on
  d : Constant  Value=disc.d
  rho : Constant  Value=amb.rho
  vector-norm : MATLAB Function  TreatAsAtomicUnit=on
  q-inf-S : Outport
  q-inf-S-d : Outport  Port=2
  wires:
  d/1 -> Product2/2
  Product2/1 -> q-inf-S-d/1
  X-to-vel/1(vel) -> vector-norm/1(vec)
  Gain/1 -> q-inf-S/1, Product2/1
  Square/1 -> Product1/1
  S/1 -> Product1/2
  vector-norm/1(norm) -> Square/1
  X/1 -> X-to-vel/1(X)
  rho/1 -> Product1/3
  Product1/1 -> Gain/1

== system hummel_and_hubbard/flatball-6dof/calc-F-M/lab/helpers/Subsystem ==
  Xdot : Inport
  Display : Display
  Gain : Gain  Gain=-1
  Ground2 : Ground
  Ground3 : Ground
  Ta1 : MATLAB Function  TreatAsAtomicUnit=on
  zero-side-slip-angle : MATLAB Function  TreatAsAtomicUnit=on
  Ta23 : Outport
  wires:
  Ground2/1 -> Ta1/2(theta)
  Gain/1 -> Ta1/3(psi)
  Ground3/1 -> Ta1/1(phi)
  Ta1/1(T) -> Ta23/1  "Ta23"
  zero-side-slip-angle/1(beta) -> Display/1, Gain/1  "beta"
  Xdot/1 -> zero-side-slip-angle/1(Xdot)

== system hummel_and_hubbard/flatball-6dof/calc-F-M/lab/helpers/Subsystem1 ==
  X1_dot : Inport
  TH1_dot : Inport  Port=2
  TH1 : Inport  Port=3
  Display : Display
  Display1 : Display
  MatrixMultiply : Product  Multiplication=Matrix(*)
  MatrixMultiply1 : Product  Multiplication=Matrix(*)
  transformation-matrices : Subsystem
  w_ : MATLAB Function  TreatAsAtomicUnit=on
  X2_dot : Outport
  TH2_dot : Outport  Port=2
  w~ : Outport  Port=3
  wires:
  MatrixMultiply/1 -> Display/1, X2_dot/1
  MatrixMultiply1/1 -> w_/1(THdot), Display1/1, TH2_dot/1
  transformation-matrices/1(Ta12) -> MatrixMultiply/1
  transformation-matrices/2(Tr12) -> MatrixMultiply1/1
  X1_dot/1 -> MatrixMultiply/2
  TH1_dot/1 -> MatrixMultiply1/2
  TH1/1 -> transformation-matrices/1(TH)
  w_/1(M) -> w~/1  "w_"

== system hummel_and_hubbard/flatball-6dof/calc-F-M/lab/helpers/Subsystem2 ==
  Xdot : Inport
  Display : Display
  Ground : Ground
  Ground1 : Ground
  Ta2 : MATLAB Function  TreatAsAtomicUnit=on
  angle-of-attack : MATLAB Function  TreatAsAtomicUnit=on
  Ta34 : Outport
  wires:
  Ground1/1 -> Ta2/3(psi)
  Ta2/1(T) -> Ta34/1  "Ta34"
  angle-of-attack/1(alpha) -> Display/1, Ta2/2(theta)  "alpha"
  Xdot/1 -> angle-of-attack/1(Xdot)
  Ground/1 -> Ta2/1(phi)

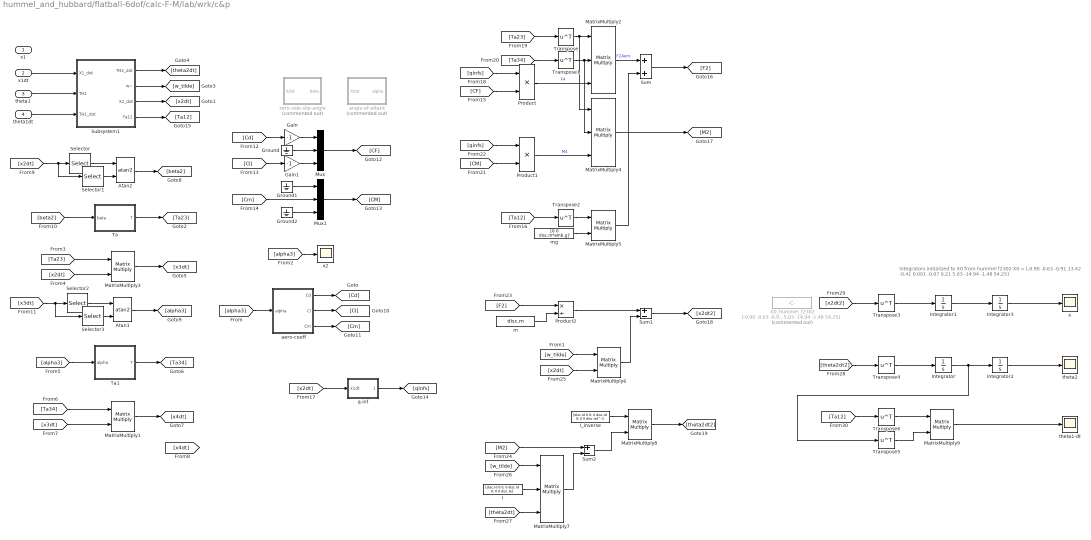
== system hummel_and_hubbard/flatball-6dof/calc-F-M/lab/wrk/c&p ==
  note: integrators initialized to X0 from hummel f2302
      | X0 = [-0.90 -0.63 -0.91 13.42 -0.41 0.001 -0.07 0.21 5.03 -14.94 -1.48 54.25]
  x1 : Inport
  x1dt : Inport  Port=2
  theta1 : Inport  Port=3
  theta1dt : Inport  Port=4
  Atan1 : Trigonometry  Operator=atan2
  Atan2 : Trigonometry  Operator=atan2
  Gain : Gain  Gain=-1
  Gain1 : Gain  Gain=-1
  Ground : Ground
  Ground1 : Ground
  Ground2 : Ground
  I : Constant  Value=[disc.Id 0 0; 0 disc.Id 0; 0 0 disc.Ia]
  I_inverse : Constant  Value=[disc.Id 0 0; 0 disc.Id 0; 0 0 disc.Ia]^-1
  Integrator : Integrator  InitialCondition=[-14.94 -1.48 54.25]
  Integrator1 : Integrator  InitialCondition=[13.42 -0.41 0.001]
  Integrator2 : Integrator  InitialCondition=[-0.07 0.21 5.03]
  Integrator3 : Integrator  InitialCondition=[-0.90 -0.63 -0.91]
  MatrixMultiply{1,3,5..6,8..9} (6 alike) : Product  Multiplication=Matrix(*)
  MatrixMultiply2 : Product  Inputs=3  Multiplication=Matrix(*)
  MatrixMultiply4 : Product  Inputs=3  Multiplication=Matrix(*)
  MatrixMultiply7 : Product  Inputs=3  Multiplication=Matrix(*)
  Mux : Mux  Inputs=3
  Mux1 : Mux  Inputs=3
  Product : Product
  Product1 : Product
  Product2 : Product  Inputs=*/
  Selector : Selector  InputPortWidth=3  IndexOptions=Index vector (dialog)  Indices=[2]  OutputSizes=1
  Selector1 : Selector  InputPortWidth=3  IndexOptions=Index vector (dialog)  Indices=[1]  OutputSizes=1
  Selector2 : Selector  InputPortWidth=3  IndexOptions=Index vector (dialog)  Indices=[3]  OutputSizes=1
  Selector3 : Selector  InputPortWidth=3  IndexOptions=Index vector (dialog)  Indices=[1]  OutputSizes=1
  Subsystem1 : Subsystem
  Sum : Sum
  Sum1 : Sum  Inputs=+-
  Sum2 : Sum  Inputs=+-
  Ta : MATLAB Function  TreatAsAtomicUnit=on
  Ta1 : MATLAB Function  TreatAsAtomicUnit=on
  Transpose{,1..6} (7 alike) : Math  Operator=transpose  SaturateOnIntegerOverflow=on
  X0_hummel_f2302 : Constant  Commented=on  Value=[-0.90 -0.63 -0.91 13.42 -0.41 0.001 -0.07 0.21 5.03 -14.94 -1.48 54.25]
  aero-coeff : Subsystem
  angle-of-attack : MATLAB Function  Commented=on  TreatAsAtomicUnit=on
  m : Constant  Value=disc.m
  mg : Constant  Value=[0 0 disc.m*amb.g]'
  q-inf : Subsystem
  theta1-dt : Scope
  theta2 : Scope
  x : Scope
  x2 : Scope
  zero-side-slip-angle : MATLAB Function  Commented=on  TreatAsAtomicUnit=on
  wires:
  x1dt/1 -> Subsystem1/1(X1_dot)
  theta1dt/1 -> Subsystem1/3(TH1_dot)
  theta1/1 -> Subsystem1/2(TH1)
  Ta/1(T) -> [Ta23]
  Subsystem1/2(w~) -> [w_tilde]
  Subsystem1/1(TH2_dot) -> [theta2dt]
  [beta2] -> Ta/1(beta)
  MatrixMultiply3/1 -> [x3dt]
  [alpha3] -> Ta1/1(alpha)
  Ta1/1(T) -> [Ta34]
  MatrixMultiply1/1 -> [x4dt]
  [x2dt] -> Selector1/1, Selector/1
  Atan2/1 -> [beta2]
  Atan1/1 -> [alpha3]
  aero-coeff/1(Cd) -> [Cd]
  aero-coeff/3(Cm) -> [Cm]
  aero-coeff/2(Cl) -> [Cl]
  [alpha3] -> aero-coeff/1(alpha)
  [Cd] -> Gain/1
  [Cl] -> Gain1/1
  Ground/1 -> Mux/2
  Mux/1 -> [CF]
  Gain/1 -> Mux/1
  Gain1/1 -> Mux/3
  [Cm] -> Mux1/2
  Ground1/1 -> Mux1/1
  Ground2/1 -> Mux1/3
  Mux1/1 -> [CM]
  [x2dt] -> q-inf/1(x1dt)
  q-inf/1(q-inf-S) -> [qinfs]
  [qinfs] -> Product/1
  [CF] -> Product/2
  [Ta34] -> Transpose1/1
  [Ta23] -> Transpose/1
  Transpose/1 -> MatrixMultiply4/1, MatrixMultiply2/1
  Transpose1/1 -> MatrixMultiply4/2, MatrixMultiply2/2
  Product/1 -> MatrixMultiply2/3  "F4"
  [CM] -> Product1/2
  [qinfs] -> Product1/1
  Product1/1 -> MatrixMultiply4/3  "M4"
  [Ta23] -> MatrixMultiply3/1
  [x2dt] -> MatrixMultiply3/2
  [x3dt] -> MatrixMultiply1/2
  [Ta34] -> MatrixMultiply1/1
  Subsystem1/4(Ta12) -> [Ta12]
  [Ta12] -> Transpose2/1
  Transpose2/1 -> MatrixMultiply5/1
  mg/1 -> MatrixMultiply5/2
  MatrixMultiply2/1 -> Sum/1  "F2Aero"
  MatrixMultiply5/1 -> Sum/2
  Sum/1 -> [F2]
  MatrixMultiply4/1 -> [M2]
  [F2] -> Product2/1
  m/1 -> Product2/2
  Product2/1 -> Sum1/1
  [w_tilde] -> MatrixMultiply6/1
  [x2dt] -> MatrixMultiply6/2
  MatrixMultiply6/1 -> Sum1/2
  Sum1/1 -> [x2dt2]
  [M2] -> Sum2/1
  [theta2dt] -> MatrixMultiply7/3
  [w_tilde] -> MatrixMultiply7/1
  I/1 -> MatrixMultiply7/2
  MatrixMultiply7/1 -> Sum2/2
  MatrixMultiply8/1 -> [theta2dt2]
  [theta2dt2] -> Transpose4/1
  [x2dt2] -> Transpose3/1
  Integrator/1 -> Integrator2/1, Transpose5/1
  Integrator1/1 -> Integrator3/1
  Integrator2/1 -> theta2/1
  Integrator3/1 -> x/1
  I_inverse/1 -> MatrixMultiply8/1
  Sum2/1 -> MatrixMultiply8/2
  Subsystem1/3(X2_dot) -> [x2dt]
  Transpose3/1 -> Integrator1/1
  Transpose4/1 -> Integrator/1
  [alpha3] -> x2/1
  Selector/1 -> Atan2/1
  Selector1/1 -> Atan2/2
  Selector3/1 -> Atan1/2
  Selector2/1 -> Atan1/1
  [x3dt] -> Selector3/1, Selector2/1
  Transpose5/1 -> MatrixMultiply9/2
  [Ta12] -> Transpose6/1
  Transpose6/1 -> MatrixMultiply9/1
  MatrixMultiply9/1 -> theta1-dt/1

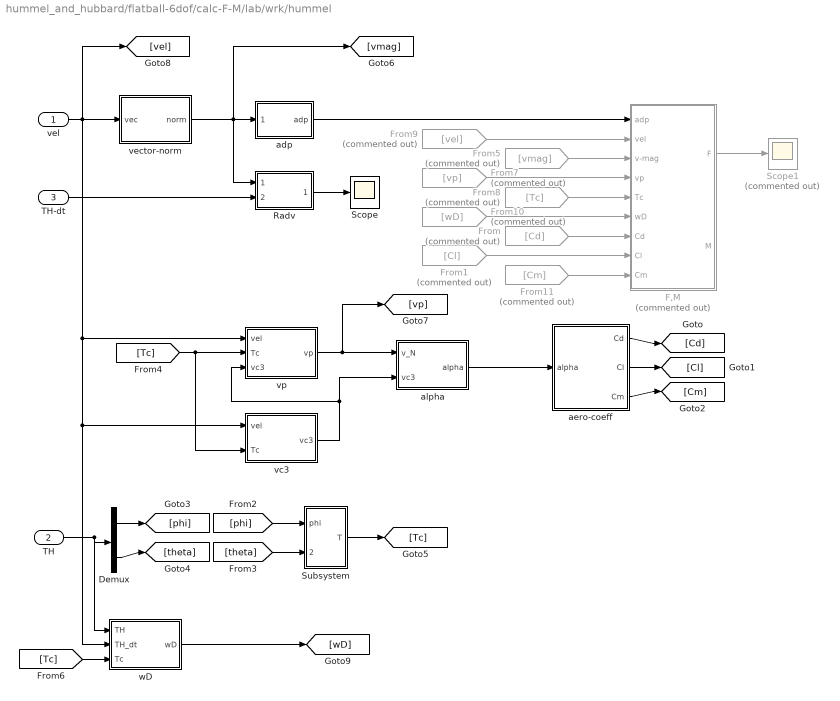
== system hummel_and_hubbard/flatball-6dof/calc-F-M/lab/wrk/hummel ==
  vel : Inport
  TH : Inport  Port=2
  TH-dt : Inport  Port=3
  Demux : Demux  Outputs=2
  F,M : Subsystem  Commented=on
  From : From  Commented=on  GotoTag=Cd
  From1 : From  Commented=on  GotoTag=Cl
  From10 : From  Commented=on  GotoTag=wD
  From11 : From  Commented=on  GotoTag=Cm
  From5 : From  Commented=on  GotoTag=vmag
  From7 : From  Commented=on  GotoTag=vp
  From8 : From  Commented=on  GotoTag=Tc
  From9 : From  Commented=on  GotoTag=vel
  Radv : Subsystem
  Scope : Scope
  Scope1 : Scope  Commented=on
  Subsystem : Subsystem
  adp : Subsystem
  aero-coeff : Subsystem
  alpha : MATLAB Function  TreatAsAtomicUnit=on
  vc3 : MATLAB Function  TreatAsAtomicUnit=on
  vector-norm : MATLAB Function  TreatAsAtomicUnit=on
  vp : MATLAB Function  TreatAsAtomicUnit=on
  wD : MATLAB Function  TreatAsAtomicUnit=on
  wires:
  aero-coeff/1(Cd) -> [Cd]
  aero-coeff/2(Cl) -> [Cl]
  aero-coeff/3(Cm) -> [Cm]
  adp/1(adp) -> F,M/1(adp)
  vel/1 -> [vel], wD/2(TH_dt), vc3/1(vel), vp/1(vel), vector-norm/1(vec)
  TH/1 -> wD/1(TH), Demux/1
  Demux/2 -> [theta]
  Demux/1 -> [phi]
  [phi] -> Subsystem/1(phi)
  [theta] -> Subsystem/2(theta)
  vector-norm/1(norm) -> Radv/1(v-mag), [vmag], adp/1(v-mag)
  Subsystem/1(T) -> [Tc]
  vp/1(vp) -> [vp], alpha/1(v_N)
  [Tc] -> vc3/2(Tc), vp/2(Tc)
  vc3/1(vc3) -> vp/3(vc3), alpha/2(vc3)
  alpha/1(alpha) -> aero-coeff/1(alpha)
  TH-dt/1 -> Radv/2(TH-dt)
  Radv/1(Radv) -> Scope/1
  [Tc] -> wD/3(Tc)
  wD/1(wD) -> [wD]
  From5/1 -> F,M/3(v-mag)
  From7/1 -> F,M/4(vp)
  From8/1 -> F,M/5(Tc)
  F,M/1(F) -> Scope1/1
  From9/1 -> F,M/2(vel)
  From10/1 -> F,M/6(wD)
  From/1 -> F,M/7(Cd)
  From1/1 -> F,M/8(Cl)
  From11/1 -> F,M/9(Cm)

== system hummel_and_hubbard/flatball-6dof/lab/work-in-progress/body-forces-and-moments/mg ==
  Constant1 : Constant  Value=amb.g
  Constant2 : Constant  Value=disc.m
  Ground4 : Ground
  Ground5 : Ground
  Mux2 : Mux  Inputs=3
  Product4 : Product
  mg : Outport
  wires:
  Ground5/1 -> Mux2/2
  Mux2/1 -> Product4/2
  Constant2/1 -> Product4/1
  Ground4/1 -> Mux2/1
  Constant1/1 -> Mux2/3
  Product4/1 -> mg/1

== system hummel_and_hubbard/flatball-6dof/lab/work-in-progress/earth-reference/beta2 ==
  X2dot : Inport
  Atan2 : Trigonometry  Operator=atan2
  Selector : Selector  InputPortWidth=3  IndexOptions=Index vector (dialog)  Indices=[2]  OutputSizes=1
  Selector3 : Selector  InputPortWidth=3  IndexOptions=Index vector (dialog)  Indices=[1]  OutputSizes=1
  tag scope: beta2=scoped
  wires:
  X2dot/1 -> Selector/1, Selector3/1
  Selector3/1 -> Atan2/2  "u2"
  Selector/1 -> Atan2/1  "v2"
  Atan2/1 -> [beta2]

== system hummel_and_hubbard/flatball-6dof/lab/work-in-progress/earth-reference/v_inf ==
  X2dot : Inport
  Demux : Demux  Outputs=3
  Sqrt : Sqrt  SaturateOnIntegerOverflow=on
  Square : Math  Operator=square  SaturateOnIntegerOverflow=on
  Square1 : Math  Operator=square  SaturateOnIntegerOverflow=on
  Square2 : Math  Operator=square  SaturateOnIntegerOverflow=on
  Sum : Sum  Inputs=3
  tag scope: v_inf=scoped
  wires:
  Sqrt/1 -> [v_inf]
  Demux/2 -> Square1/1
  X2dot/1 -> Demux/1
  Demux/3 -> Square2/1
  Square/1 -> Sum/1
  Demux/1 -> Square/1
  Sum/1 -> Sqrt/1
  Square2/1 -> Sum/3
  Square1/1 -> Sum/2

== system hummel_and_hubbard/flatball-6dof/lab/work-in-progress/earth-reference/w_tilde ==
  X2dot : Inport
  MATLAB Function : MATLAB Function  TreatAsAtomicUnit=on
  tag scope: w_tilde=scoped
  wires:
  X2dot/1 -> MATLAB Function/1(X2dot)
  MATLAB Function/1(w) -> [w_tilde]
